simulink model "N_scheme_RS_unstructured"  (R2024b)
settings: Solver=VariableStepAuto  StartTime=0.0  StopTime=10.0  RelTol=1e-3
values from neighbouring files (symbols this model uses):
  Ga = 0.01    [p14.m]
  Gf = 1/(Kd*Gs)    (= 0.166666666667)    [p14.m]
  Gs = 1    [p14.m]
libraries: cstblocks x3
settings Model: Creator=adrian  LastModifiedBy=adrian

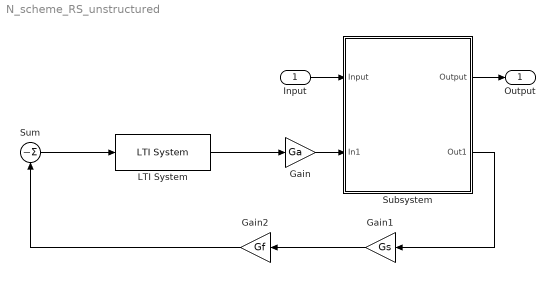
== system N_scheme_RS_unstructured ==
  Input : Inport
  Gain : Gain  Gain=Ga
  Gain1 : Gain  Gain=Gs
  Gain2 : Gain  Gain=Gf
  LTI System : cstblocks/LTI System  sys=Gc  IC=[]  PadeOrder=0
  Subsystem : Subsystem
  Sum : Sum  Inputs=|-
  Output : Outport
  wires:
  LTI System/1 -> Gain/1
  Gain1/1 -> Gain2/1
  Sum/1 -> LTI System/1
  Gain/1 -> Subsystem/2(In1)
  Subsystem/2(Out1) -> Gain1/1
  Input/1 -> Subsystem/1(Input)
  Subsystem/1(Output) -> Output/1
  Gain2/1 -> Sum/1

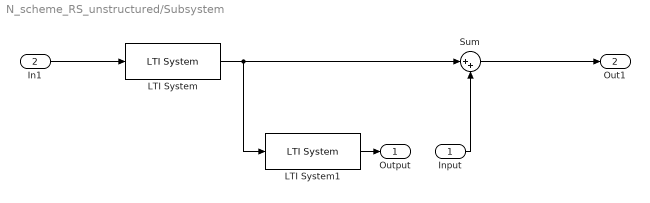
== system N_scheme_RS_unstructured/Subsystem ==
  Input : Inport
  In1 : Inport  Port=2
  LTI System : cstblocks/LTI System  sys=Gpn  IC=[]  PadeOrder=0
  LTI System1 : cstblocks/LTI System  sys=Wu_new  IC=[]  PadeOrder=0
  Sum : Sum  Inputs=|++
  Output : Outport
  Out1 : Outport  Port=2
  wires:
  In1/1 -> LTI System/1
  LTI System/1 -> Sum/1, LTI System1/1
  Input/1 -> Sum/2
  Sum/1 -> Out1/1
  LTI System1/1 -> Output/1
